simulink model "thermo_openloop_v2"  (R2018b)
settings: Solver=VariableStepAuto  StartTime=0.0  StopTime=10.0  RelTol=1e-3
undefined symbols (not defined in the file or in its folder): baud, com, fTf, fTl, fTt, input_fan, input_lamp, input_led, Ts
libraries: tos_lib x1

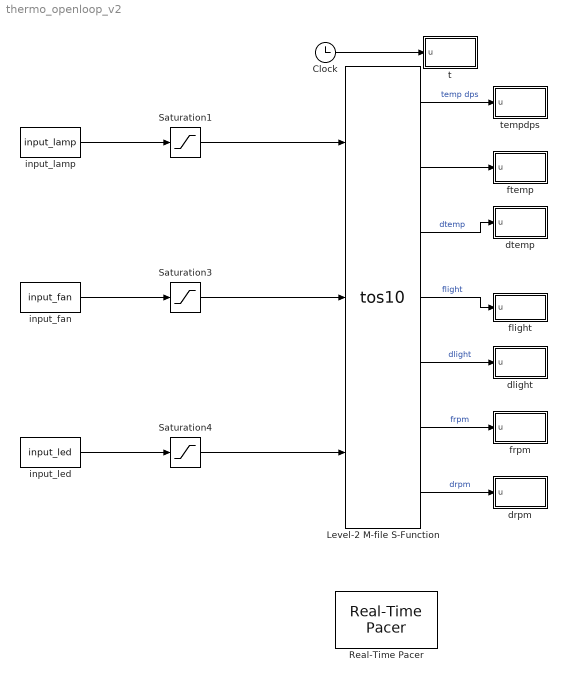
== system thermo_openloop_v2 ==
  Clock : Clock
  Level-2 M-file S-Function : M-S-Function  FunctionName=tos10  Parameters=Ts,com,baud,fTt,fTl,fTf
  Real-Time Pacer : tos_lib/Real-Time Pacer  simTimePerRealTime=1
  Saturation1 : Saturate  UpperLimit=100  LowerLimit=0  SampleTime=Ts
  Saturation3 : Saturate  UpperLimit=100  LowerLimit=0  SampleTime=Ts
  Saturation4 : Saturate  UpperLimit=100  LowerLimit=0  SampleTime=Ts
  dlight : MATLAB Function  TreatAsAtomicUnit=on  SystemSampleTime=Ts
  drpm : MATLAB Function  TreatAsAtomicUnit=on  SystemSampleTime=Ts
  dtemp : MATLAB Function  TreatAsAtomicUnit=on  SystemSampleTime=Ts
  flight : MATLAB Function  TreatAsAtomicUnit=on  SystemSampleTime=Ts
  frpm : MATLAB Function  TreatAsAtomicUnit=on  SystemSampleTime=Ts
  ftemp : MATLAB Function  TreatAsAtomicUnit=on  SystemSampleTime=Ts
  input_fan : Constant  Value=input_fan  SampleTime=Ts
  input_lamp : Constant  Value=input_lamp  SampleTime=Ts
  input_led : Constant  Value=input_led  SampleTime=Ts
  t : MATLAB Function  TreatAsAtomicUnit=on  SystemSampleTime=Ts
  tempdps : MATLAB Function  TreatAsAtomicUnit=on  SystemSampleTime=Ts
  wires:
  Level-2 M-file S-Function/6 -> frpm/1(u)  "frpm"
  Saturation1/1 -> Level-2 M-file S-Function/1
  Level-2 M-file S-Function/5 -> dlight/1(u)  "dlight"
  Saturation3/1 -> Level-2 M-file S-Function/2
  Level-2 M-file S-Function/2 -> ftemp/1(u)
  Clock/1 -> t/1(u)
  Level-2 M-file S-Function/7 -> drpm/1(u)  "drpm"
  input_led/1 -> Saturation4/1
  Level-2 M-file S-Function/4 -> flight/1(u)  "flight"
  Level-2 M-file S-Function/3 -> dtemp/1(u)  "dtemp"
  Level-2 M-file S-Function/1 -> tempdps/1(u)  "temp dps"
  Saturation4/1 -> Level-2 M-file S-Function/3
  input_lamp/1 -> Saturation1/1
  input_fan/1 -> Saturation3/1

== matlab function thermo_openloop_v2/ftemp ==
  data: u input
function fcn(u)
%#eml
eml.extrinsic('num2str');
eml.extrinsic('strcat');
eml.extrinsic('evalin');
evalin('base',strcat('ftemp(end+1)=', num2str(u),';'));
end

== matlab function thermo_openloop_v2/tempdps ==
  data: u input
function fcn(u)
%#eml
eml.extrinsic('num2str');
eml.extrinsic('strcat');
eml.extrinsic('evalin');
evalin('base',strcat('tempdps(end+1)=', num2str(u),';'));
end

== matlab function thermo_openloop_v2/dtemp ==
  data: u input
function fcn(u)
%#eml
eml.extrinsic('num2str');
eml.extrinsic('strcat');
eml.extrinsic('evalin');
evalin('base',strcat('dtemp(end+1)=', num2str(u),';'));
end

== matlab function thermo_openloop_v2/frpm ==
  data: u input
function fcn(u)
%#eml
eml.extrinsic('num2str');
eml.extrinsic('strcat');
eml.extrinsic('evalin');
evalin('base',strcat('frpm(end+1)=', num2str(u),';'));
end

== matlab function thermo_openloop_v2/drpm ==
  data: u input
function fcn(u)
%#eml
eml.extrinsic('num2str');
eml.extrinsic('strcat');
eml.extrinsic('evalin');
evalin('base',strcat('drpm(end+1)=', num2str(u),';'));
end

== matlab function thermo_openloop_v2/flight ==
  data: u input
function fcn(u)
%#eml
eml.extrinsic('num2str');
eml.extrinsic('strcat');
eml.extrinsic('evalin');
evalin('base',strcat('flight(end+1)=', num2str(u),';'));
end

== matlab function thermo_openloop_v2/dlight ==
  data: u input
function fcn(u)
%#eml
eml.extrinsic('num2str');
eml.extrinsic('strcat');
eml.extrinsic('evalin');
evalin('base',strcat('dlight(end+1)=', num2str(u),';'));
end

== matlab function thermo_openloop_v2/t ==
  data: u input
function fcn(u)
%#eml
eml.extrinsic('num2str');
eml.extrinsic('strcat');
eml.extrinsic('evalin');
evalin('base',strcat('t(end+1)=', num2str(u),';'));
end
